simulink model "test"  (R2012b)
settings: Solver=FixedStepDiscrete  StartTime=0.0  StopTime=inf  RelTol=1e-3
libraries: MAVLink_Block x1
settings Model: Creator=fede  LastModifiedBy=fede

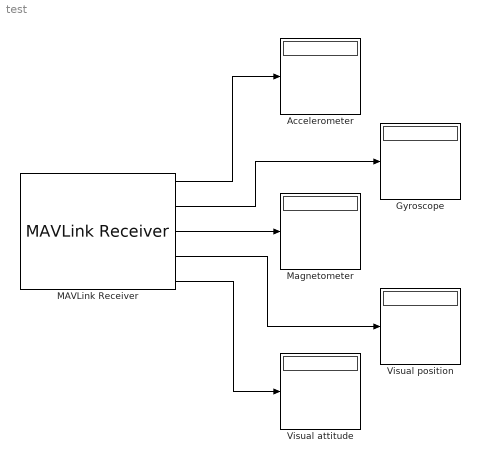
== system test ==
  Accelerometer : Display
  Gyroscope : Display
  MAVLink Receiver : MAVLink_Block/MAVLink Receiver  Port=14550  FS=1  accel=on  gyro=on  magn=on  vispos=on  visatt=on  msg_vector=0
  Magnetometer : Display
  Visual attitude : Display
  Visual position : Display
  wires:
  MAVLink Receiver/2 -> Gyroscope/1
  MAVLink Receiver/1 -> Accelerometer/1
  MAVLink Receiver/5 -> Visual attitude/1
  MAVLink Receiver/4 -> Visual position/1
  MAVLink Receiver/3 -> Magnetometer/1
